simulink model "Motor_Control"  (R2022a)
settings: Solver=FixedStepAuto  StartTime=0.0  StopTime=10.0  FixedStep=Ts  RelTol=1e-3
values from neighbouring files (symbols this model uses):
  P = 2    [Motor_Para.m]
  Ts = 1/10000    (= 0.0001)    [Motor_Para.m]
  Vbus = 24    [Motor_Para.m]
libraries: simulink x2, mcbplantlib x1, autolibpmsmexterior x1
settings Model: Creator=hp  LastModifiedBy=hp

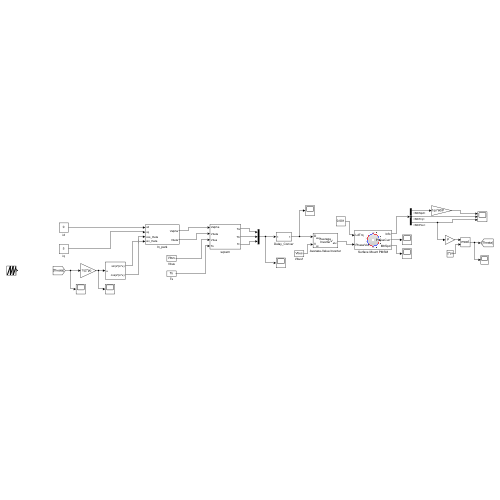
[thumbnail: Simulink's stored preview of the top-level diagram]
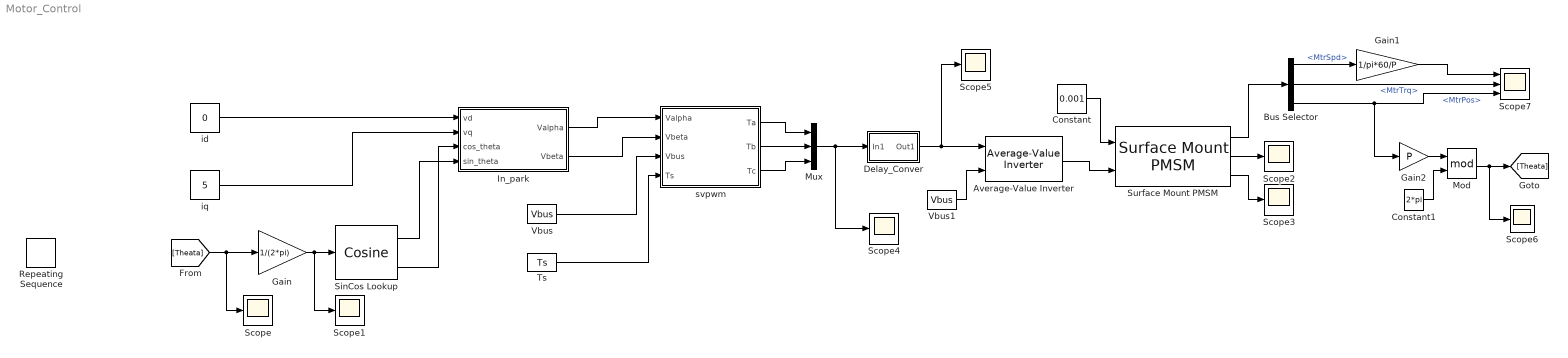
== system Motor_Control ==
  Average-Value Inverter : mcbplantlib/Average-Value Inverter
  Bus Selector : BusSelector  OutputSignals=MtrSpd,MtrTrq,MtrPos
  Constant : Constant  Value=0.001
  Constant1 : Constant  Value=2*pi
  Delay_Conver : Subsystem
  Gain : Gain  Gain=1/(2*pi)
  Gain1 : Gain  Gain=1/pi*60/P
  Gain2 : Gain  Gain=P
  In_park : Subsystem
  Mod : Math  Operator=mod
  Mux : Mux  Inputs=3
  Repeating Sequence : simulink/Sources/Repeating Sequence  rep_seq_t=[0 1/20]  rep_seq_y=[0 2*pi]
  Scope{,1..6} (7 alike) : Scope
  Scope7 : Scope  NumInputPorts=3
  SinCos Lookup : simulink/Lookup Tables/Cosine  Formula=sin(2*pi*u) and cos(2*pi*u)  NumDataPoints=(2^5)+1  OutputWordLength=16  InternalRulePriority=Speed
      settings: SourceProductBaseCode=SL
  Surface Mount PMSM : autolibpmsmexterior/Surface Mount PMSM  port_config=Torque  sim_type=Continuous  Ts=0.001  FilePath=E:\Sandbox\Bauto\Work\surfacepmsm_motordata.m  P=P  Rs=Rs  Ldq_=Ls  KConstText=Permanent flux linkage constant (lambda_pm):  lambda_pm=Flux  Ke=159.9771  Kt=1.323  mechanical=[0.00001, 4.924e-5, 0]  idq0=[0 0]  theta_init=0  omega_init=0  KConst=Flux  lambda_pm_calc=Flux  RefBlkName='autolibpmsmexterior/Surface Mount PMSM'  aMode=1  Ldq="[0.0003752   0.0003752]"
      settings: SourceProductBaseCode=PW,DR,MT,VE
  Ts : Constant  Value=Ts
  Vbus : Constant  Value=Vbus
  Vbus1 : Constant  Value=Vbus
  id : Constant  Value=0
  iq : Constant  Value=5
  svpwm : Subsystem
  wires:
  Gain/1 -> Scope1/1, SinCos Lookup/1
  id/1 -> In_park/1(vd)
  iq/1 -> In_park/2(vq)
  SinCos Lookup/1 -> In_park/4(sin_theta)
  SinCos Lookup/2 -> In_park/3(cos_theta)
  In_park/1(Valpha) -> svpwm/1(Valpha)
  In_park/2(Vbeta) -> svpwm/2(Vbeta)
  Vbus/1 -> svpwm/3(Vbus)
  Ts/1 -> svpwm/4(Ts)
  Vbus1/1 -> Average-Value Inverter/2
  Average-Value Inverter/1 -> Surface Mount PMSM/2
  Constant/1 -> Surface Mount PMSM/1
  svpwm/2(Tb) -> Mux/2
  svpwm/1(Ta) -> Mux/1
  svpwm/3(Tc) -> Mux/3
  Surface Mount PMSM/2 -> Scope2/1
  Surface Mount PMSM/3 -> Scope3/1
  Mux/1 -> Scope4/1, Delay_Conver/1(In1)
  Delay_Conver/1(Out1) -> Scope5/1, Average-Value Inverter/1
  Surface Mount PMSM/1 -> Bus Selector/1
  Bus Selector/3 -> Gain2/1, Scope7/3  "<MtrPos>"
  Bus Selector/2 -> Scope7/2  "<MtrTrq>"
  Bus Selector/1 -> Gain1/1  "<MtrSpd>"
  Gain1/1 -> Scope7/1
  Gain2/1 -> Mod/1
  Mod/1 -> Scope6/1, [Theata]
  Constant1/1 -> Mod/2
  [Theata] -> Scope/1, Gain/1

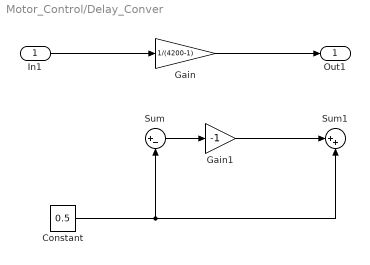
== system Motor_Control/Delay_Conver ==
  In1 : Inport
  Constant : Constant  Value=0.5
  Gain : Gain  Gain=1/(4200-1)
  Gain1 : Gain  Gain=-1
  Sum : Sum  Inputs=|+-
  Sum1 : Sum  Inputs=|++
  Out1 : Outport
  wires:
  In1/1 -> Gain/1
  Constant/1 -> Sum1/2, Sum/2
  Sum/1 -> Gain1/1
  Gain1/1 -> Sum1/1
  Gain/1 -> Out1/1

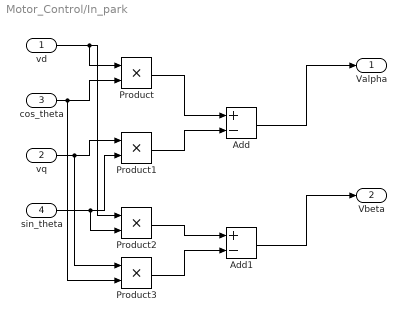
== system Motor_Control/In_park ==
  vd : Inport
  vq : Inport  Port=2
  cos_theta : Inport  Port=3
  sin_theta : Inport  Port=4
  Add : Sum  Inputs=+-
  Add1 : Sum  Inputs=+-
  Product{,1..3} (4 alike) : Product
  Valpha : Outport
  Vbeta : Outport  Port=2
  wires:
  vd/1 -> Product2/1, Product/1
  cos_theta/1 -> Product3/2, Product/2
  vq/1 -> Product3/1, Product1/1
  sin_theta/1 -> Product2/2, Product1/2
  Product/1 -> Add/1
  Product1/1 -> Add/2
  Add/1 -> Valpha/1
  Product2/1 -> Add1/1
  Product3/1 -> Add1/2
  Add1/1 -> Vbeta/1

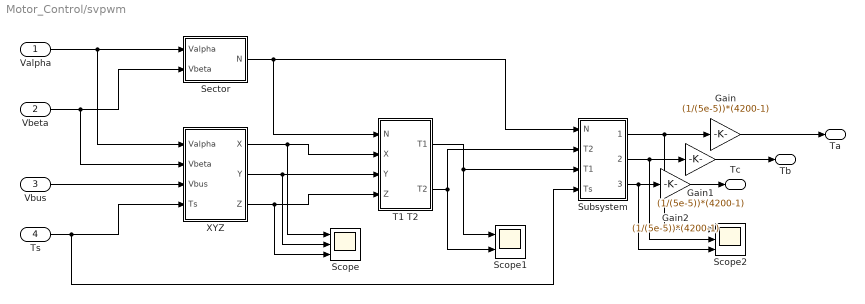
== system Motor_Control/svpwm ==
  Valpha : Inport
  Vbeta : Inport  Port=2
  Vbus : Inport  Port=3
  Ts : Inport  Port=4
  Gain : Gain  Gain=(1/(5e-5))*(4200-1)
  Gain1 : Gain  Gain=(1/(5e-5))*(4200-1)
  Gain2 : Gain  Gain=(1/(5e-5))*(4200-1)
  Scope : Scope  NumInputPorts=3
  Scope1 : Scope  NumInputPorts=2
  Scope2 : Scope  NumInputPorts=3
  Sector : Subsystem
  Subsystem : Subsystem
  T1 T2 : Subsystem
  XYZ : Subsystem
  Ta : Outport
  Tb : Outport  Port=2
  Tc : Outport  Port=3
  wires:
  Valpha/1 -> XYZ/1(Valpha), Sector/1(Valpha)
  Vbeta/1 -> XYZ/2(Vbeta), Sector/2(Vbeta)
  Vbus/1 -> XYZ/3(Vbus)
  Ts/1 -> Subsystem/4(Ts), XYZ/4(Ts)
  XYZ/1(X) -> Scope/1, T1 T2/2(X)
  XYZ/2(Y) -> Scope/2, T1 T2/3(Y)
  XYZ/3(Z) -> Scope/3, T1 T2/4(Z)
  Sector/1(N) -> Subsystem/1(N), T1 T2/1(N)
  T1 T2/1(T1) -> Subsystem/3(T1), Scope1/1
  T1 T2/2(T2) -> Subsystem/2(T2), Scope1/2
  Subsystem/2(Tcm2) -> Scope2/2, Gain1/1
  Subsystem/1(Tcm1) -> Scope2/1, Gain/1
  Subsystem/3(Tcm3) -> Scope2/3, Gain2/1
  Gain/1 -> Ta/1
  Gain1/1 -> Tb/1
  Gain2/1 -> Tc/1

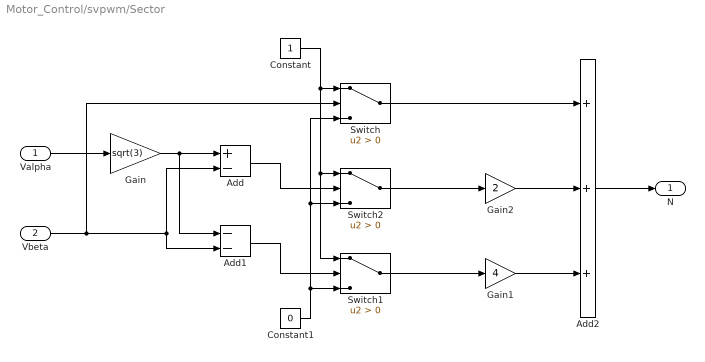
== system Motor_Control/svpwm/Sector ==
  Valpha : Inport
  Vbeta : Inport  Port=2
  Add : Sum  Inputs=+-
  Add1 : Sum  Inputs=--
  Add2 : Sum  Inputs=+++
  Constant : Constant
  Constant1 : Constant  Value=0
  Gain : Gain  Gain=sqrt(3)
  Gain1 : Gain  Gain=4
  Gain2 : Gain  Gain=2
  Switch : Switch  Criteria=u2 > Threshold  SaturateOnIntegerOverflow=off  InputSameDT=off
  Switch1 : Switch  Criteria=u2 > Threshold  SaturateOnIntegerOverflow=off  InputSameDT=off
  Switch2 : Switch  Criteria=u2 > Threshold  SaturateOnIntegerOverflow=off  InputSameDT=off
  N : Outport
  wires:
  Valpha/1 -> Gain/1
  Gain/1 -> Add1/1, Add/1
  Vbeta/1 -> Switch/2, Add1/2, Add/2
  Constant/1 -> Switch1/1, Switch2/1, Switch/1
  Constant1/1 -> Switch1/3, Switch/3, Switch2/3
  Add/1 -> Switch2/2
  Add1/1 -> Switch1/2
  Switch1/1 -> Gain1/1
  Switch2/1 -> Gain2/1
  Switch/1 -> Add2/1
  Gain2/1 -> Add2/2
  Gain1/1 -> Add2/3
  Add2/1 -> N/1

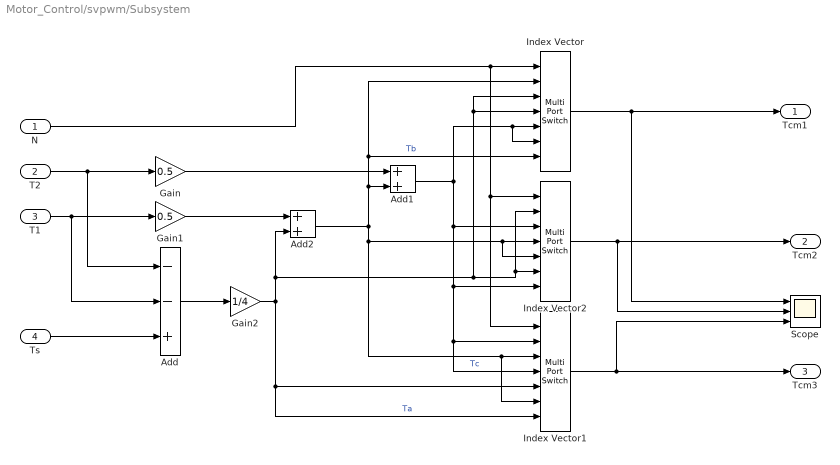
== system Motor_Control/svpwm/Subsystem ==
  N : Inport
  T2 : Inport  Port=2
  T1 : Inport  Port=3
  Ts : Inport  Port=4
  Add : Sum  Inputs=--+
  Add1 : Sum
  Add2 : Sum
  Gain : Gain  Gain=0.5
  Gain1 : Gain  Gain=0.5
  Gain2 : Gain  Gain=1/4
  Index Vector : MultiPortSwitch  Inputs=6  SaturateOnIntegerOverflow=off  InputSameDT=off
  Index Vector1 : MultiPortSwitch  Inputs=6  SaturateOnIntegerOverflow=off  InputSameDT=off
  Index Vector2 : MultiPortSwitch  Inputs=6  SaturateOnIntegerOverflow=off  InputSameDT=off
  Scope : Scope  NumInputPorts=3
  Tcm1 : Outport
  Tcm2 : Outport  Port=2
  Tcm3 : Outport  Port=3
  wires:
  T2/1 -> Add/1, Gain/1
  T1/1 -> Add/2, Gain1/1
  Ts/1 -> Add/3
  Add/1 -> Gain2/1
  Gain2/1 -> Index Vector1/7, Index Vector1/5, Index Vector/4, Index Vector/3, Index Vector2/6, Index Vector2/2, Add2/2  "Ta"
  Gain1/1 -> Add2/1
  Add2/1 -> Index Vector2/5, Index Vector2/4, Index Vector1/6, Index Vector1/3, Index Vector/2, Index Vector/7, Add1/2  "Tb"
  Gain/1 -> Add1/1
  N/1 -> Index Vector1/1, Index Vector2/1, Index Vector/1
  Index Vector/1 -> Scope/1, Tcm1/1
  Index Vector2/1 -> Scope/2, Tcm2/1
  Index Vector1/1 -> Scope/3, Tcm3/1
  Add1/1 -> Index Vector/6, Index Vector/5, Index Vector2/3, Index Vector2/7, Index Vector1/4, Index Vector1/2  "Tc"

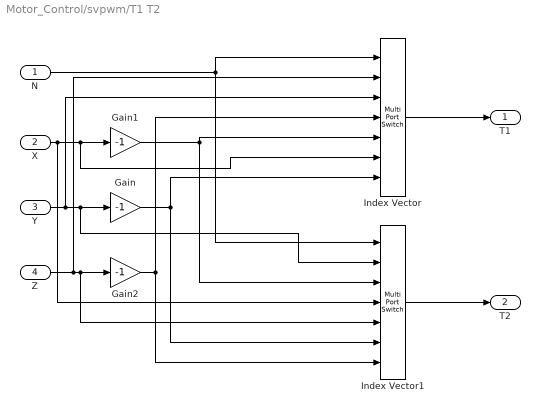
== system Motor_Control/svpwm/T1 T2 ==
  N : Inport
  X : Inport  Port=2
  Y : Inport  Port=3
  Z : Inport  Port=4
  Gain : Gain  Gain=-1
  Gain1 : Gain  Gain=-1
  Gain2 : Gain  Gain=-1
  Index Vector : MultiPortSwitch  Inputs=6  SaturateOnIntegerOverflow=off  InputSameDT=off
  Index Vector1 : MultiPortSwitch  Inputs=6  SaturateOnIntegerOverflow=off  InputSameDT=off
  T1 : Outport
  T2 : Outport  Port=2
  wires:
  X/1 -> Gain1/1, Index Vector/6, Index Vector1/4
  Y/1 -> Gain/1, Index Vector1/2, Index Vector/3
  Z/1 -> Index Vector1/5, Gain2/1, Index Vector/2
  Index Vector/1 -> T1/1
  Index Vector1/1 -> T2/1
  N/1 -> Index Vector1/1, Index Vector/1
  Gain1/1 -> Index Vector1/3, Index Vector/5
  Gain2/1 -> Index Vector1/7, Index Vector/4
  Gain/1 -> Index Vector/7, Index Vector1/6

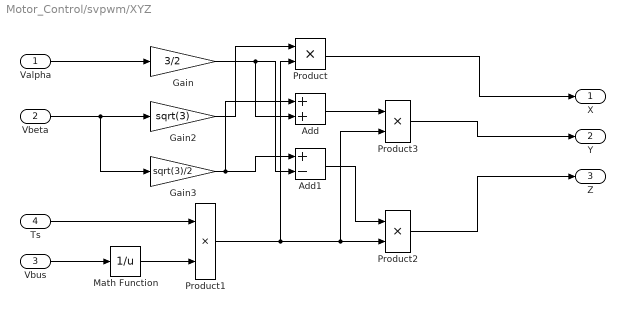
== system Motor_Control/svpwm/XYZ ==
  Valpha : Inport
  Vbeta : Inport  Port=2
  Vbus : Inport  Port=3
  Ts : Inport  Port=4
  Add : Sum
  Add1 : Sum  Inputs=+-
  Gain : Gain  Gain=3/2
  Gain2 : Gain  Gain=sqrt(3)
  Gain3 : Gain  Gain=sqrt(3)/2
  Math Function : Math  Operator=reciprocal
  Product{,1..3} (4 alike) : Product
  X : Outport
  Y : Outport  Port=2
  Z : Outport  Port=3
  wires:
  Valpha/1 -> Gain/1
  Vbeta/1 -> Gain3/1, Gain2/1
  Gain/1 -> Add1/2, Add/2
  Gain2/1 -> Product/1
  Vbus/1 -> Math Function/1
  Math Function/1 -> Product1/2
  Ts/1 -> Product1/1
  Gain3/1 -> Add/1, Add1/1
  Product1/1 -> Product3/2, Product2/2, Product/2
  Add1/1 -> Product2/1
  Add/1 -> Product3/1
  Product2/1 -> Z/1
  Product3/1 -> Y/1
  Product/1 -> X/1
